simulink model "LAFES_FRFIvan"  (R2024a)
settings: Solver=FixedStepAuto  StartTime=0.0  StopTime=3600  FixedStep=0.01  RelTol=1e-3
PreLoadFcn:
  | addpath(genpath('./S_Functions'))
  | run('model.m')
InitFcn:
  | NETIF =  'eth0';
model workspace (MAT data in the model file):
  ENC_LINK_ID = 1
  SWITCH_LINK_ID = 1
  collocated = Simulink.Parameter
  collocated.Value = 1
  collocated.Complexity = 'real'
  collocated.Dimensions = [1 1]
  collocated.DataType = 'boolean'
  fb_hardware = Simulink.Parameter
  fb_hardware.Value = 1
  fb_hardware.Complexity = 'real'
  fb_hardware.Dimensions = [1 1]
  fb_hardware.DataType = 'boolean'
  link_id = 1
  system_enable = Simulink.Parameter
  system_enable.Value = 0
  system_enable.Complexity = 'real'
  system_enable.Dimensions = [1 1]
  system_enable.DataType = 'boolean'
  use_gen_ref = Simulink.Parameter
  use_gen_ref.Value = 0
  use_gen_ref.Complexity = 'real'
  use_gen_ref.Dimensions = [1 1]
  use_gen_ref.DataType = 'boolean'
  zero_follower = Simulink.Parameter
  zero_follower.Value = 0
  zero_follower.Complexity = 'real'
  zero_follower.Dimensions = [1 1]
  zero_follower.DataType = 'boolean'
  zero_leader = Simulink.Parameter
  zero_leader.Value = 0
  zero_leader.Complexity = 'real'
  zero_leader.Dimensions = [1 1]
  zero_leader.DataType = 'boolean'
libraries: simulink x2, slctrl_linear x1
settings Model: SimulationMode=external  Creator=20192648  LastModifiedBy=20201350
settings HardwareCC: ProdBitPerLong=64  ProdHWDeviceType=Intel->x86-64 (Linux 64)
settings ModelReferenceCC: EnableRefExpFcnMdlSchedulingChecks=on  PropagateSignalLabelsOutOfModel=off
settings RTWCC: Description=RoboCup Realtime Target  SystemTargetFile=mttarget.tlc  MakeCommand="make_rtw CC=\"ccache gcc\" OPTS=\"-DNETIF_ID=0 -DTEST_CONN_MODEL -D_GNU_SOURCE -DPRIO=99\""  TemplateMakefile=mt_unix.tmf  CustomInclude=./S_Functions  RTWCompilerOptimization=Custom  RTWCustomCompilerOptimizations=-O2 -g -W
settings RTWCC: CustomSource=|
  | Rs485EthercatLibrary.c
  | ethercatbase.c
  | ethercatcoe.c
  | ethercatconfig.c
  | ethercatdc.c
  | ethercatfoe.c
  | ethercatmain.c
  | ethercatprint.c
  | ethercatsoe.c
  | nicdrv.c
  | osal.c
  | oshw.c
  | timer_posix.c
  | timer_stats.c
settings CodeAppCC: StateflowObjectComments=on
settings GRTTargetCC: TargetLangStandard=C89/C90 (ANSI)  CodeReplacementLibrary=GNU C99 extensions  UseToolchainInfoCompliant=off  ExtMode=on

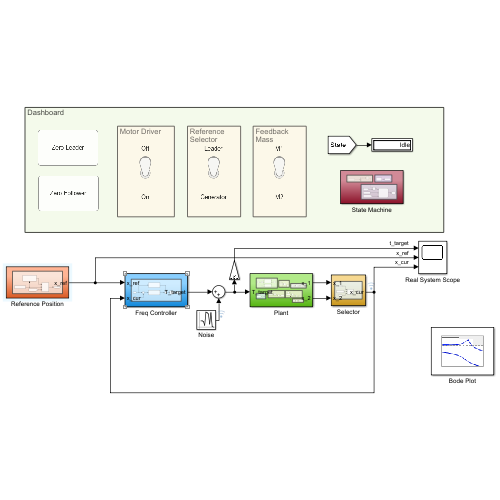
[thumbnail: Simulink's stored preview of the top-level diagram]
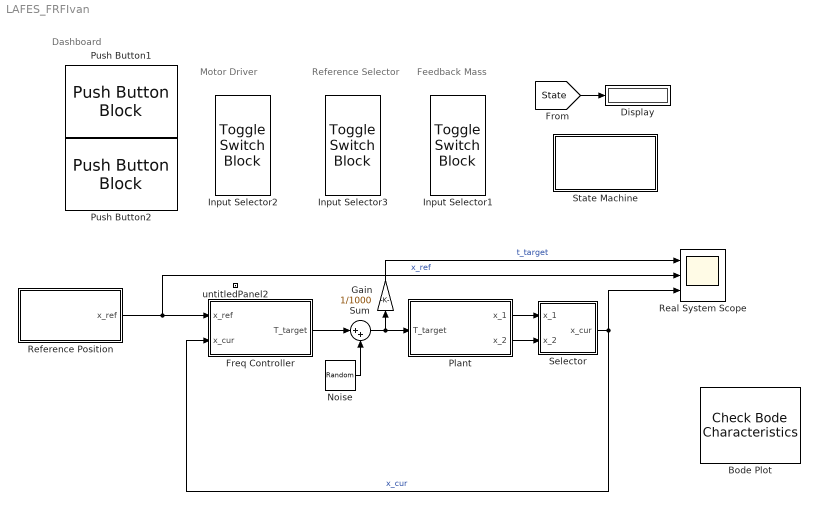
== system LAFES_FRFIvan ==
  note: Dashboard
  note: Reference
      | Selector
  note: Motor Driver
  note: Feedback
      | Mass
  Bode Plot : slctrl_linear/Check Bode  Characteristics  InstantiateOnLoad=on  SaveOperatingPoints=off  LinearizationIOs={}  LinearizeAt=SnapshotTimes  SnapshotTimes=[0]  TriggerType=rising  SampleTime=auto  RateConversionMethod=zoh  PreWarpFreq=10  UseExactDelayModel=off  UseFullBlockNameLabels=off  UseBusSignalLabels=off  enabled=on  stopWhenAssertionFail=off  export=off  ViewDlgPos=[]  OpenViewOnLoad=off  LaunchViewOnOpen=off  FrequencyUnits=rad/s  MagnitudeUnits=dB  PhaseUnits=deg  TimeUnits=seconds  EnableUpperBound=off  UpperBoundFrequencies=[]  UpperBoundMagnitudes=[]  EnableLowerBound=off  LowerBoundFrequencies=[]  LowerBoundMagnitudes=[]
      settings: LibrarySourceBlock=slctrlblks/Linear Analysis Plots/Bode Plot  SaveToWorkspace=off  SaveName=sys
  Display : Display
  Freq Controller : Subsystem
  Gain : Gain  Gain=1/1000
  Input Selector1 : ToggleSwitchBlock  LabelPosition=Hide
      settings: Values={{'M2', 'M1'}, [0 1]}
  Input Selector2 : ToggleSwitchBlock  LabelPosition=Hide
      settings: Values={{'On', 'Off'}, [1 0]}
  Input Selector3 : ToggleSwitchBlock  LabelPosition=Hide
      settings: Values={{'Generator', 'Leader'}, [1 0]}
  Noise : RandomNumber  Variance=0.1  SampleTime=250
  Plant : Subsystem
  Push Button1 : PushButtonBlock  ButtonText=Zero Leader  OffValue=0.000000
  Push Button2 : PushButtonBlock  ButtonText=Zero Follower  OffValue=0.000000
  Real System Scope : Scope  NumInputPorts=3
  Reference Position : Subsystem
  Selector : Subsystem
  State Machine : Subsystem
  Sum : Sum  Inputs=|++
  untitledPanel2 : Subsystem  Tag=HiddenForWebPanel  IsWebBlockPanel=on
  wires:
  Plant/1(x_1) -> Selector/1(x_1)
  Plant/2(x_2) -> Selector/2(x_2)
  Reference Position/1(x_ref) -> Freq Controller/1(x_ref), Real System Scope/2  "x_ref"
  Gain/1 -> Real System Scope/1  "t_target"
  [State] -> Display/1
  Selector/1(x_cur) -> Freq Controller/2(x_cur), Real System Scope/3  "x_cur"
  Freq Controller/1(T_target) -> Sum/1
  Sum/1 -> Gain/1, Plant/1(T_target)
  Noise/1 -> Sum/2

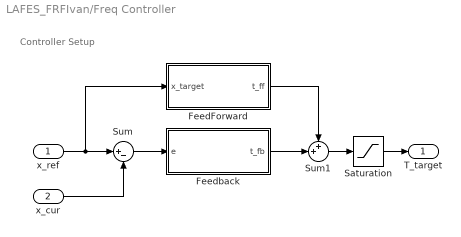
== system LAFES_FRFIvan/Freq Controller ==
  note: Controller Setup
  x_ref : Inport
  x_cur : Inport  Port=2
  FeedForward : Subsystem
  Feedback : Subsystem
  Saturation : Saturate  UpperLimit=1000  LowerLimit=-1000
  Sum : Sum  Inputs=|+-
  Sum1 : Sum  Inputs=++|
  T_target : Outport
  wires:
  FeedForward/1(t_ff) -> Sum1/1
  Feedback/1(t_fb) -> Sum1/2
  Sum1/1 -> Saturation/1
  x_ref/1 -> FeedForward/1(x_target), Sum/1
  Sum/1 -> Feedback/1(e)
  x_cur/1 -> Sum/2
  Saturation/1 -> T_target/1

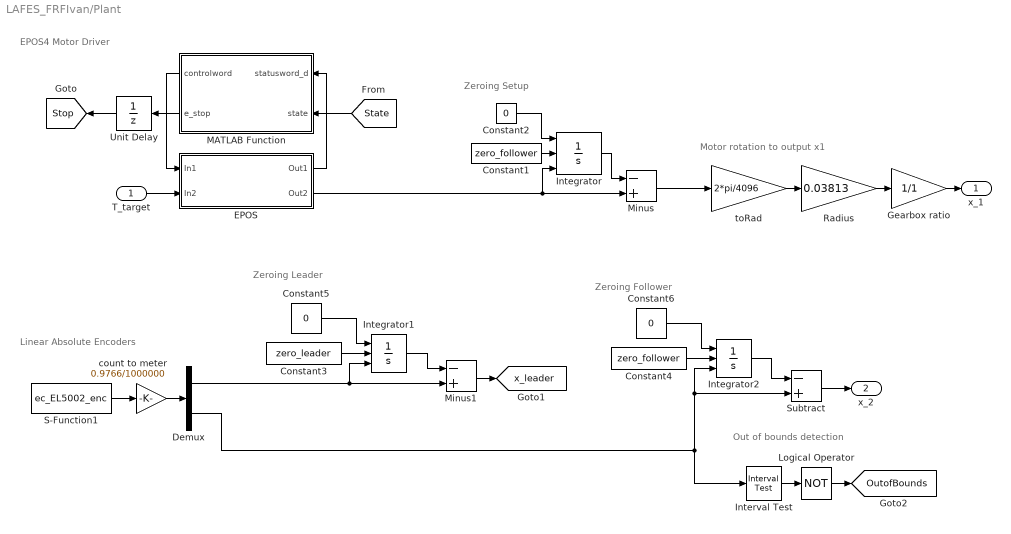
== system LAFES_FRFIvan/Plant ==
  note: Linear Absolute Encoders
  note: Zeroing Follower
  note: Zeroing Leader
  note: Zeroing Setup
  note: Motor rotation to output x1
  note: EPOS4 Motor Driver
  note: Out of bounds detection
  T_target : Inport
  Constant1 : Constant  Value=zero_follower
  Constant2 : Constant  Value=0
  Constant3 : Constant  Value=zero_leader
  Constant4 : Constant  Value=zero_follower
  Constant5 : Constant  Value=0
  Constant6 : Constant  Value=0
  Demux : Demux  Outputs=2
  EPOS : Subsystem  mask{link_id=1, operating_mode=CyclicSynchronousTorque}
      mask prompts: link_id "link id > 0"; operating_mode "Operating mode of the drive"
      mask TypeOptions operating_mode: CyclicSynchronousPosition | CyclicSynchronousVelocity | CyclicSynchronousTorque
  Gearbox ratio : Gain  Gain=1/1
  Integrator : Integrator  ExternalReset=rising  InitialConditionSource=external
  Integrator1 : Integrator  ExternalReset=rising  InitialConditionSource=external
  Integrator2 : Integrator  ExternalReset=rising  InitialConditionSource=external
  Interval Test : simulink/Logic and Bit Operations/Interval Test  IntervalClosedRight=on  uplimit=15.07  IntervalClosedLeft=on  lowlimit=14.04  OutDataTypeStr=boolean
  Logical Operator : Logic  Operator=NOT  AllPortsSameDT=off  OutDataTypeStr=boolean
  MATLAB Function : MATLAB Function  TreatAsAtomicUnit=on
  Minus : Sum  Inputs=-+
  Minus1 : Sum  Inputs=-+
  Radius : Gain  Gain=0.03813
  S-Function1 : S-Function  FunctionName=ec_EL5002_enc  Parameters=ENC_LINK_ID  SFunctionDeploymentMode=off  EnableBusSupport=off
  Subtract : Sum  Inputs=-+
  Unit Delay : UnitDelay  SampleTime=-1  HasFrameUpgradeWarning=on
  count to meter : Gain  Gain=0.9766/1000000
  toRad : Gain  Gain=2*pi/4096
  x_1 : Outport
  x_2 : Outport  Port=2
  tag scope: OutofBounds=global, Stop=global, x_leader=global
  wires:
  [State] -> MATLAB Function/2(state)
  Unit Delay/1 -> [Stop]
  MATLAB Function/1(controlword) -> EPOS/1(In1)
  Integrator/1 -> Minus/1
  EPOS/2(Out2) -> Integrator/3, Minus/2
  Constant2/1 -> Integrator/1
  Constant1/1 -> Integrator/2
  Minus/1 -> toRad/1
  Gearbox ratio/1 -> x_1/1
  EPOS/1(Out1) -> MATLAB Function/1(statusword_d)
  MATLAB Function/2(e_stop) -> Unit Delay/1
  T_target/1 -> EPOS/2(In2)
  Radius/1 -> Gearbox ratio/1
  toRad/1 -> Radius/1
  Logical Operator/1 -> [OutofBounds]
  Subtract/1 -> x_2/1
  Integrator2/1 -> Subtract/1
  Integrator1/1 -> Minus1/1
  Constant6/1 -> Integrator2/1
  Constant3/1 -> Integrator1/2
  Constant4/1 -> Integrator2/2
  S-Function1/1 -> count to meter/1
  Constant5/1 -> Integrator1/1
  Interval Test/1 -> Logical Operator/1
  Minus1/1 -> [x_leader]
  count to meter/1 -> Demux/1
  Demux/1 -> Integrator1/3, Minus1/2
  Demux/2 -> Interval Test/1, Subtract/2, Integrator2/3

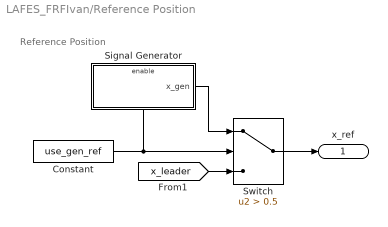
== system LAFES_FRFIvan/Reference Position ==
  note: Reference Position
  Constant : Constant  Value=use_gen_ref
  Signal Generator : Subsystem  TreatAsAtomicUnit=on
  Switch : Switch  Criteria=u2 > Threshold  Threshold=0.5  SaturateOnIntegerOverflow=off  InputSameDT=off
  x_ref : Outport
  wires:
  [x_leader] -> Switch/3
  Constant/1 -> Signal Generator/Enable, Switch/2
  Switch/1 -> x_ref/1
  Signal Generator/1(x_gen) -> Switch/1

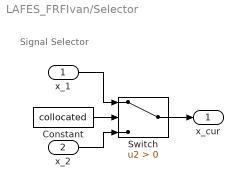
== system LAFES_FRFIvan/Selector ==
  note: Signal Selector
  x_1 : Inport
  x_2 : Inport  Port=2
  Constant : Constant  Value=collocated
  Switch : Switch  Criteria=u2 > Threshold  SaturateOnIntegerOverflow=off  InputSameDT=off
  x_cur : Outport
  wires:
  Switch/1 -> x_cur/1
  Constant/1 -> Switch/2
  x_1/1 -> Switch/1
  x_2/1 -> Switch/3

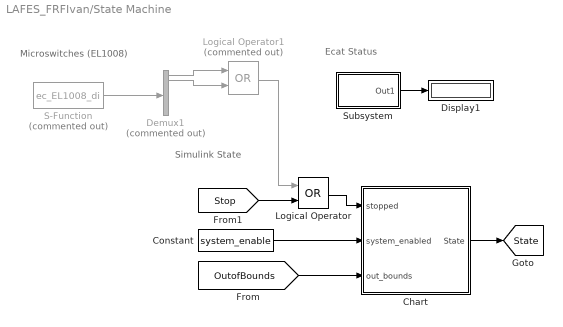
== system LAFES_FRFIvan/State Machine ==
  note: Simulink State
  note: Ecat Status
  note: Microswitches (EL1008)
  Chart : Stateflow chart  TreatAsAtomicUnit=on
  Constant : Constant  Value=system_enable  OutDataTypeStr=boolean
  Demux1 : Demux  Commented=on  Outputs=8
  Display1 : Display
  Logical Operator : Logic  Operator=OR  AllPortsSameDT=off  OutDataTypeStr=boolean
  Logical Operator1 : Logic  Commented=on  Operator=OR  AllPortsSameDT=off
  S-Function : S-Function  Commented=on  FunctionName=ec_EL1008_di  Parameters=SWITCH_LINK_ID  SFunctionDeploymentMode=off  EnableBusSupport=off
  Subsystem : Subsystem  mask{NETIF=NETIF}
  tag scope: State=global
  wires:
  [OutofBounds] -> Chart/3(out_bounds)
  Chart/1(State) -> [State]
  Constant/1 -> Chart/2(system_enabled)
  [Stop] -> Logical Operator/2
  Demux1/1 -> Logical Operator1/1
  Logical Operator1/1 -> Logical Operator/1
  Demux1/2 -> Logical Operator1/2
  S-Function/1 -> Demux1/1
  Subsystem/1(Out1) -> Display1/1
  Logical Operator/1 -> Chart/1(stopped)

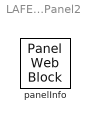
== system LAFES_FRFIvan/untitledPanel2 ==
  panelInfo : PanelWebBlock  Tag=HiddenForWebPanel  PanelInfo="{\"compacted\":false,\"height\":250,\"isActiveTab\":true,\"left\":209,\"name\":\"Panel2\",\"panelId\":\"panelId-2b300b07-a086-47ad-816e-87b5706ef90b\",\"popoutData\":{\"height\":0,\"left\":0,\"maximized\":false,\"top\":0,\"width\":0},\"popoutMode\":\"componentHidden\",\"tabIndex\":0,\"tabbedSetId\":\"tabbedSet4045690118\",\"top\":404,\"type\":\"panel\",\"version\":\"2019b\",\"visible\":true,\"width\":250,\"zIndex\":1500006}"  PanelSnapshot=<binary blob, 700 chars, not shown>

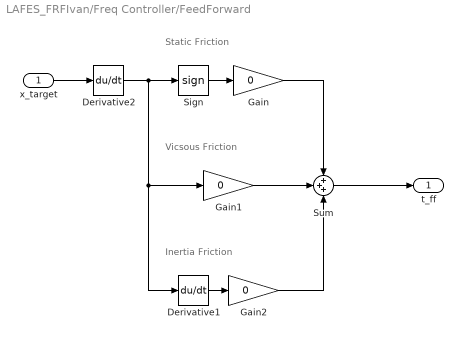
== system LAFES_FRFIvan/Freq Controller/FeedForward ==
  note: Inertia Friction
  note: Vicsous Friction
  note: Static Friction
  x_target : Inport
  Derivative1 : Derivative
  Derivative2 : Derivative
  Gain : Gain  Gain=0
  Gain1 : Gain  Gain=0
  Gain2 : Gain  Gain=0
  Sign : Signum
  Sum : Sum  Inputs=+++
  t_ff : Outport
  wires:
  x_target/1 -> Derivative2/1
  Sign/1 -> Gain/1
  Derivative1/1 -> Gain2/1
  Gain/1 -> Sum/1
  Gain1/1 -> Sum/2
  Gain2/1 -> Sum/3
  Sum/1 -> t_ff/1
  Derivative2/1 -> Gain1/1, Derivative1/1, Sign/1

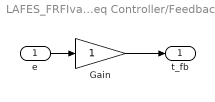
== system LAFES_FRFIvan/Freq Controller/Feedback ==
  e : Inport
  Gain : Gain
  t_fb : Outport
  wires:
  e/1 -> Gain/1
  Gain/1 -> t_fb/1

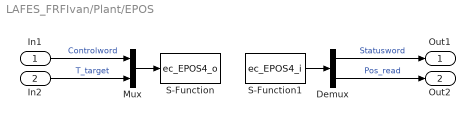
== system LAFES_FRFIvan/Plant/EPOS ==
  In1 : Inport
  In2 : Inport  Port=2
  Demux : Demux  Outputs=2
  Mux : Mux  Inputs=2
  S-Function : S-Function  FunctionName=ec_EPOS4_o  Parameters=link_id  SFunctionDeploymentMode=off  EnableBusSupport=off
  S-Function1 : S-Function  FunctionName=ec_EPOS4_i  Parameters=link_id operating_mode  SFunctionDeploymentMode=off  EnableBusSupport=off
  Out1 : Outport
  Out2 : Outport  Port=2
  wires:
  In1/1 -> Mux/1  "Controlword"
  In2/1 -> Mux/2  "T_target"
  Mux/1 -> S-Function/1
  S-Function1/1 -> Demux/1
  Demux/1 -> Out1/1  "Statusword"
  Demux/2 -> Out2/1  "Pos_read"

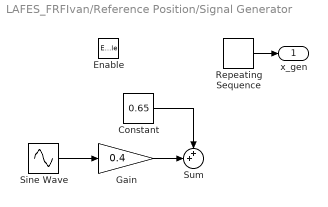
== system LAFES_FRFIvan/Reference Position/Signal Generator ==
  Enable : EnablePort
  Constant : Constant  Value=0.65
  Gain : Gain  Gain=0.4
  Repeating Sequence : simulink/Sources/Repeating Sequence  rep_seq_t=[0 5 10 15 20]  rep_seq_y=[0 80 0 -80 0]
  Sine Wave : Sin  Frequency=5  SampleTime=0
  Sum : Sum  Inputs=++|
  x_gen : Outport
  wires:
  Sine Wave/1 -> Gain/1
  Gain/1 -> Sum/2
  Constant/1 -> Sum/1
  Repeating Sequence/1 -> x_gen/1

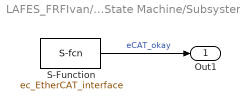
== system LAFES_FRFIvan/State Machine/Subsystem ==
  S-Function : S-Function  FunctionName=ec_EtherCAT_interface  Parameters=NETIF  SFunctionDeploymentMode=off  EnableBusSupport=off
  Out1 : Outport
  wires:
  S-Function/1 -> Out1/1  "eCAT_okay"

== matlab function LAFES_FRFIvan/Plant/MATLAB Function ==
  data: statusword_d input; controlword output; state input; e_stop output
function [controlword, e_stop] = fcn(statusword_d, state)

%% === Statusword bits ===
BIT_READY_TO_SWITCH_ON    = uint16(1);
BIT_SWITCHED_ON           = uint16(2);
BIT_OPERATION_ENABLED     = uint16(4);
BIT_FAULT                 = uint16(8);
BIT_QUICK_STOP            = uint16(32);
BIT_SWITCH_ON_DISABLED    = uint16(64);

%% === Controlwords ===
CTRL_SHUTDOWN     = uint16(6);
CTRL_SWITCH_ON    = uint16(7);
CTRL_ENABLE_OP    = uint16(15);
CTRL_QUICK_STOP   = uint16(2);
CTRL_FAULT_RESET  = uint16(128);

%% Convert raw statusword
statusword = uint16(statusword_d);

%% === Correct hardware E-STOP detection ===
estop_active = bitand(statusword, BIT_SWITCH_ON_DISABLED) ~= 0;

% Hardware estop only if switch_on_disabled active and YOU were running
e_stop = estop_active && ...
         state == SystemStateEnum.Running;

%% === Priority 1: Hardware ESTOP ===
if e_stop
    controlword = double(CTRL_SHUTDOWN);
    return;
end

switch state
    % === Priority 2: Logical STOP from supervisor ===
    case SystemStateEnum.Stopped
        controlword = double(CTRL_SHUTDOWN);
        return

    % === Priority 3: Idle → shutdown ===
    case state == SystemStateEnum.Idle
        controlword = double(CTRL_SHUTDOWN);
        return;

    % === Priority 4: Quick stop request ===
    case state == SystemStateEnum.Out_of_Bounds
        controlword = double(CTRL_QUICK_STOP);
        return;        
end

%% === Priority 5: Running → follow CiA-402 state machine ===
if state == SystemStateEnum.Running

    if bitand(statusword, BIT_FAULT) ~= 0
        controlword = double(CTRL_FAULT_RESET);

    elseif bitand(statusword, BIT_READY_TO_SWITCH_ON) ~= 0 && ...
           bitand(statusword, BIT_SWITCHED_ON) == 0
        controlword = double(CTRL_SWITCH_ON);

    elseif bitand(statusword, BIT_SWITCHED_ON) ~= 0 && ...
           bitand(statusword, BIT_OPERATION_ENABLED) == 0
        controlword = double(CTRL_ENABLE_OP);

    elseif bitand(statusword, BIT_OPERATION_ENABLED) ~= 0
        controlword = double(CTRL_ENABLE_OP);

    else
        controlword = double(CTRL_SHUTDOWN);
    end

    return;
end

%% === Fallback ===
controlword = double(CTRL_SHUTDOWN);
end

== stateflow chart LAFES_FRFIvan/State Machine/Chart ==
  settings: sampleTime=0.01  executeAtInitialization=1
  state Not_Stopped
    state Idle
    state Running
    state Out_of_Bounds
    (default) -> Idle
    Not_Stopped -> Idle [order 1] : [~system_enabled]
    Idle -> Running : [system_enabled]
    Out_of_Bounds -> Running : [~out_bounds]
    Running -> Out_of_Bounds : [out_bounds]
  state Stopped
  (default) -> Not_Stopped
  Stopped -> Not_Stopped : [~stopped & ~system_enabled]
  Not_Stopped -> Stopped [order 1] : [stopped]
  data: stopped input; State output Enum: SystemStateEnum; system_enabled input; out_bounds input
